simulink model "test09"  (R2021a)
settings: Solver=VariableStepAuto  StartTime=0.0  StopTime=10  RelTol=1e-3
values from neighbouring files (symbols this model uses):
  crop_params = crop_p    [test09_script.m]
libraries: HORTISIM x11
settings Model: Creator=djoroya  LastModifiedBy=djoroya
settings DebuggingCC: UnconnectedInputMsg=none  UnconnectedOutputMsg=none  UnconnectedLineMsg=none

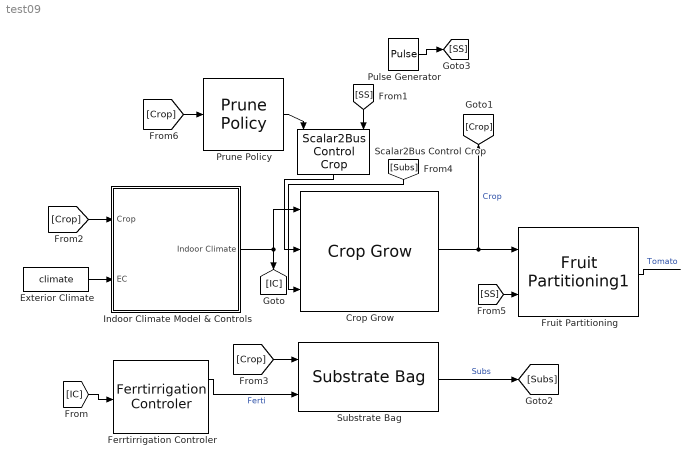
== system test09 ==
  Crop Grow : HORTISIM/Horticulture/Models/Crop Grow  Chi_nutrients="[ 0.0156    0.0104    0.0052    0.0021    0.0021    0.0010         0         0]'"  A_v=2080  plants_density=2.1562  fraction_DM=0.08  min_water_capacity=0.1  C_buf_max=0.02  T_v_start_fruit=1100  int_air_speed=0.5  b_N_uptake=0.5  Tv=288  C=crop_params.C  R=[0 0 0]  Tsum=0  C_wv=0.2  N=[0 0 0 0 0 0 0 0]'  rg_fruit=2e-7  c_fruit_m=2.3e-7  c_fruit_g=0.27  rg_leaf=9.5000e-08  c_leaf_m=3.4700e-07  c_leaf_g=0.28  rg_stem=7.4000e-08  c_stem_m=1.47e-7  c_stem_g=0.3  VelocityAbsortion=10  T_max_v=40  s_max_T=0.5793  s_min_T=-0.8690  s_buforg_buf=-5000  T_sum_end=1035  T_max_v24=27  T_min_v24=14  s_min_T24=-1.1587  s_max_T24=1.3904  T_min_v=6
      settings: SourceProductName=Horti Simulator
  Exterior Climate : FromWorkspace  VariableName=climate
  Ferrtirrigation Controler : HORTISIM/Horticulture/Controls/Ferrtirrigation  Controler  hour0=1  IrrigationFlow=1e-3  Xnutrients="1e-3*0.13*[1.0000    0.6667    0.3333    0.1333    0.1333    0.0667         0         0]"  percent_irrigation=5  Irrigation_jules_to_hours=0.5*1e-6
      settings: SourceProductName=Horti Simulator
  Fruit Partitioning : HORTISIM/Horticulture/Models/Fruit Partitioning1  Cfruit0=1e-3
      settings: SourceProductName=Horti Simulator
  Indoor Climate Model & Controls : Subsystem
  Prune Policy : HORTISIM/Horticulture/Controls/Prune Policy  SystemSampleTime=-1  VariantActivationTime=update diagram  Latency=0  AutoFrameSizeCalculation=off
      settings: SourceProductName=Horti Simulator
      mask Display: image('$imagefile'); % Use "Edit Image" on toolstrip to change.
  Pulse Generator : DiscretePulseGenerator  PulseType=Time based  Period=3  PulseWidth=50
  Scalar2Bus Control Crop : HORTISIM/Other  Functions/Scalar2Bus Control Crop  SystemSampleTime=-1  VariantActivationTime=update diagram  Latency=0  AutoFrameSizeCalculation=off
      settings: SourceProductName=Horti Simulator
  Substrate Bag : HORTISIM/Horticulture/Models/Substrate Bag  Vmax_subs=10  Vmin_subs=0.1  Nmin_subs=1e-6  C_ws=0.1  N=[0 0 0 0 0 0 0 0 ]' + 1e-5  DraingeConst=1e-3  sigma_max=1  sigma_min=1
      settings: SourceProductName=Horti Simulator
  wires:
  Indoor Climate Model & Controls/1(Indoor Climate) -> [IC], Crop Grow/1
  Crop Grow/1 -> [Crop], Fruit Partitioning/1  "Crop"
  [Crop] -> Substrate Bag/1
  Substrate Bag/1 -> [Subs]  "Subs"
  [Subs] -> Crop Grow/3
  Ferrtirrigation Controler/1 -> Substrate Bag/2  "Ferti"
  Fruit Partitioning/1 -> ?  "Tomato"
  Scalar2Bus Control Crop/1 -> Crop Grow/2
  Prune Policy/1 -> Scalar2Bus Control Crop/1
  [Crop] -> Prune Policy/1
  [Crop] -> Indoor Climate Model & Controls/1(Crop)
  Exterior Climate/1 -> Indoor Climate Model & Controls/2(EC)
  [IC] -> Ferrtirrigation Controler/1
  Pulse Generator/1 -> [SS]
  [SS] -> Scalar2Bus Control Crop/4
  [SS] -> Fruit Partitioning/2

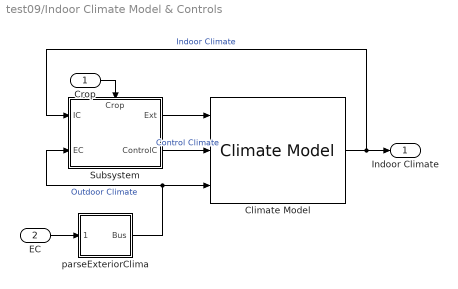
== system test09/Indoor Climate Model & Controls ==
  Crop : Inport
  EC : Inport  Port=2
  Climate Model : HORTISIM/Climate/Models/Climate Model  hour0=0  G0=[0.05 0.0007]  T0=[273 273 273 273]+15  H=7  A_f=3200  A_c=3200  minWindows=0.1  lam_s=[2.5000 0.8500]  c_s=[1081 1081]  l_s=[0.1000 0.1000]  rhod_s=[2600 2500]  int_air_speed=0.5  alpha_i=0.1  alpha_c=0.05  tau_c=0.9  alpha_f=0.1  d_c=1.5  cd_c=8736  T_ss=285.15
      settings: SourceProductName=Horti Simulator
      mask Display: image('$imagefile'); % Use "Edit Image" on toolstrip to change.
  Subsystem : Subsystem
      settings: PortSchema="{\"entries\":[{\"content\":{\"sides\":[{\"content\":{\"connectorIds\":[\"In1\",\"In2\"]},\"type\":\"ConnectorPlacement.EquallySpacedRectSide\",\"uuid\":\"05a20284-31f0-4954-ac42-b08c051c723b\"},{\"content\":{\"connectorIds\":[\"Out1\",\"Out2\"],\"side\":\"RIGHT\"},\"type\":\"ConnectorPlacement.EquallySpacedRectSide\",\"uuid\":\"7e4ab434-6629-473e-82a5-f81f17f0ab6e\"},{\"content\":{\"connectorIds\":[\"In3\"],\"side\":\"TOP\"},\"type\":\"ConnectorPlacement.EquallySpacedRectSide\",\"uuid\":\"2ea64524-8947-456a-a977-2c05776eabaa\"}]},\"type\":\"ConnectorPlacement.EquallySpacedConnector\",\"uuid\":\"6035ded9-300f-4f3c-adde-f9d2e7ea6cf9\"}],\"packageUris\":[\"http://schema.mathworks.com/mf0/Connector/R2020b\"],\"version\":\"1.0\"}"
  parseExteriorClima : Subsystem  AncestorBlock="HORTISIM/Other  Functions/parseExteriorClima"
  Indoor Climate : Outport
  wires:
  EC/1 -> parseExteriorClima/1(Array)
  Crop/1 -> Subsystem/3(Crop)
  Subsystem/2(ControlC) -> Climate Model/2  "Control Climate"
  Subsystem/1(Ext) -> Climate Model/1
  Climate Model/1 -> Subsystem/1(IC), Indoor Climate/1  "Indoor Climate"
  parseExteriorClima/1(Bus) -> Climate Model/3, Subsystem/2(EC)  "Outdoor Climate"

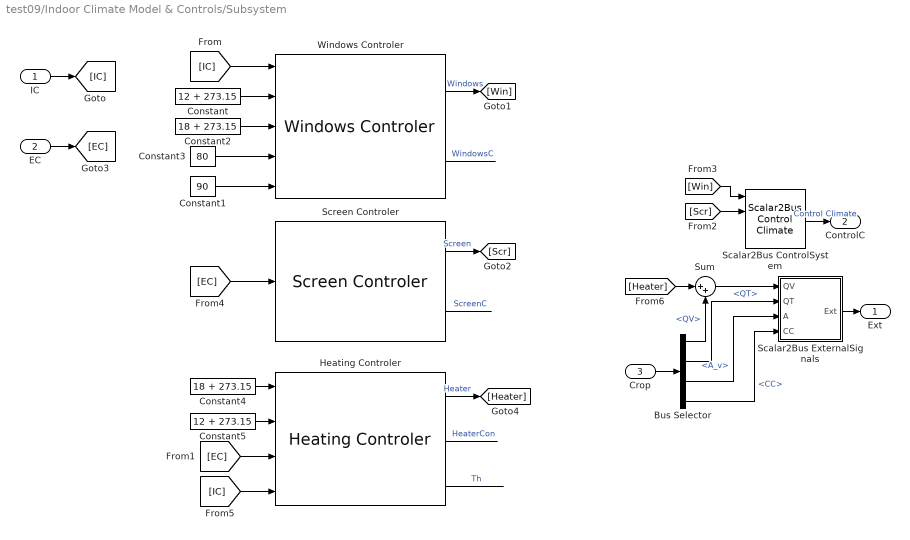
== system test09/Indoor Climate Model & Controls/Subsystem ==
  IC : Inport
  EC : Inport  Port=2
  Crop : Inport  Port=3
  Bus Selector : BusSelector  OutputSignals=HeatVars.QV,HeatVars.QT,A_v,CC
  Constant : Constant  Value=12 + 273.15
  Constant1 : Constant  Value=90
  Constant2 : Constant  Value=18 + 273.15
  Constant3 : Constant  Value=80
  Constant4 : Constant  Value=18 + 273.15
  Constant5 : Constant  Value=12 + 273.15
  Heating Controler : HORTISIM/Climate/Controls/Heating Controler  T=288  power=1000e3  A_e=6e-4  A_i=6e-4  c=1e-8
      settings: SourceProductName=Horti Simulator
  Scalar2Bus ControlSystem : HORTISIM/Other  Functions/Scalar2Bus  Control Climate  SystemSampleTime=-1  VariantActivationTime=update diagram  Latency=0  AutoFrameSizeCalculation=off
      settings: SourceProductName=Horti Simulator
  Scalar2Bus ExternalSignals : Subsystem
  Screen Controler : HORTISIM/Climate/Controls/Screen Controler  Radthreshold=200  velocity=0.33333  Power=0  gamma_max=0.3  beta=0.1
      settings: SourceProductName=Horti Simulator
  Sum : Sum  Inputs=|++
  Windows Controler : HORTISIM/Climate/Controls/Windows Controler  Power=100  max_night=10  tau=600  RadThreshold=10  AR=10
      settings: SourceProductName=Horti Simulator
  Ext : Outport
  ControlC : Outport  Port=2
  wires:
  Constant2/1 -> Windows Controler/3
  Constant3/1 -> Windows Controler/4
  Windows Controler/2 -> ?  "WindowsC"
  Constant1/1 -> Windows Controler/5
  Constant/1 -> Windows Controler/2
  IC/1 -> [IC]
  [IC] -> Windows Controler/1
  Windows Controler/1 -> [Win]  "Windows"
  Screen Controler/1 -> [Scr]  "Screen"
  [Scr] -> Scalar2Bus ControlSystem/2
  [Win] -> Scalar2Bus ControlSystem/1
  Scalar2Bus ControlSystem/1 -> ControlC/1  "Control Climate"
  EC/1 -> [EC]
  [EC] -> Screen Controler/1
  Screen Controler/2 -> ?  "ScreenC"
  [EC] -> Heating Controler/3
  [IC] -> Heating Controler/4
  Constant4/1 -> Heating Controler/1
  Constant5/1 -> Heating Controler/2
  Heating Controler/1 -> [Heater]  "Heater"
  Scalar2Bus ExternalSignals/1(Ext) -> Ext/1
  Heating Controler/3 -> ?  "Th"
  Heating Controler/2 -> ?  "HeaterCon"
  Crop/1 -> Bus Selector/1
  Bus Selector/2 -> Scalar2Bus ExternalSignals/2(QT)  "<QT>"
  [Heater] -> Sum/1
  Sum/1 -> Scalar2Bus ExternalSignals/1(QV)
  Bus Selector/1 -> Sum/2  "<QV>"
  Bus Selector/3 -> Scalar2Bus ExternalSignals/3(A)  "<A_v>"
  Bus Selector/4 -> Scalar2Bus ExternalSignals/4(CC)  "<CC>"

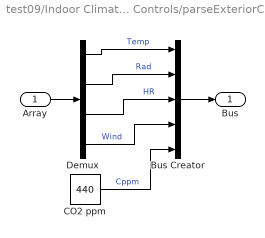
== system test09/Indoor Climate Model & Controls/parseExteriorClima ==
  Array : Inport
  Bus Creator : BusCreator  Inputs=5
  CO2 ppm : Constant  Value=440
  Demux : Demux
  Bus : Outport
  wires:
  Demux/2 -> Bus Creator/2  "Rad"
  Demux/1 -> Bus Creator/1  "Temp"
  Demux/3 -> Bus Creator/3  "HR"
  Array/1 -> Demux/1
  Demux/4 -> Bus Creator/4  "Wind"
  Bus Creator/1 -> Bus/1
  CO2 ppm/1 -> Bus Creator/5  "Cppm"

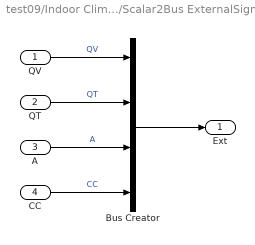
== system test09/Indoor Climate Model & Controls/Subsystem/Scalar2Bus ExternalSignals ==
  QV : Inport
  QT : Inport  Port=2
  A : Inport  Port=3
  CC : Inport  Port=4
  Bus Creator : BusCreator  Inputs=4
  Ext : Outport
  wires:
  QT/1 -> Bus Creator/2  "QT"
  QV/1 -> Bus Creator/1  "QV"
  A/1 -> Bus Creator/3  "A"
  CC/1 -> Bus Creator/4  "CC"
  Bus Creator/1 -> Ext/1
